simulink model "task3"  (R2023b)
settings: Solver=FixedStepDiscrete  StartTime=0.0  StopTime=10.0  FixedStep=5e-5  RelTol=1e-3
PreLoadFcn:
  | Simulink.defineIntEnumType('windowCommand', {'Off','Speed1','Speed2','Speed3'},[0,1,2,3])
undefined symbols (not defined in the file or in its folder): DiscIntNeverNeededParam, windowCommand
settings Model: Creator=kz1nz0  LastModifiedBy=Zuzia

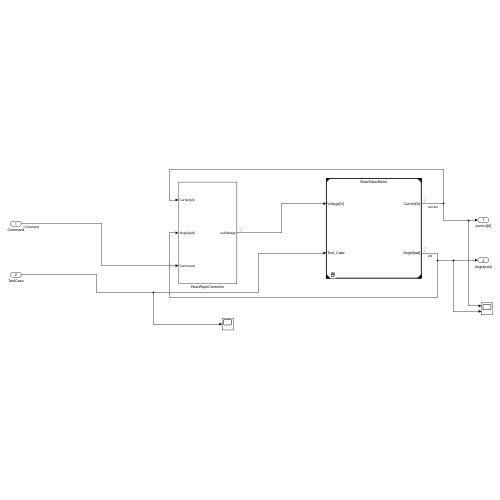
[thumbnail: Simulink's stored preview of the top-level diagram]
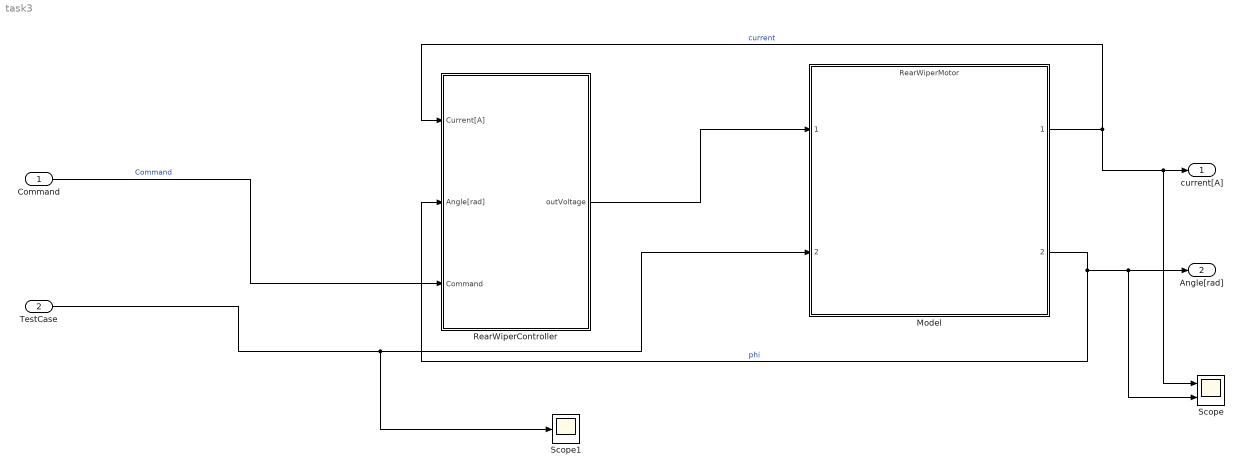
== system task3 ==
  Command : Inport  OutDataTypeStr=Enum: windowCommand
  TestCase : Inport  Port=2  OutDataTypeStr=int8
  Model : ModelReference  ModelNameDialog=RearWiperMotor.slxp  ModelReferenceVersion=19.15  CopyOfModelProtected=on
  RearWiperController : Subsystem
  Scope : Scope  NumInputPorts=2
  Scope1 : Scope
  current[A] : Outport
  Angle[rad] : Outport  Port=2
  wires:
  Command/1 -> RearWiperController/3(Command)  "Command"
  TestCase/1 -> Scope1/1, Model/2
  Model/1 -> Scope/1, current[A]/1, RearWiperController/1(Current[A])  "current"
  Model/2 -> RearWiperController/2(Angle[rad]), Scope/2, Angle[rad]/1  "phi"
  RearWiperController/1(outVoltage) -> Model/1

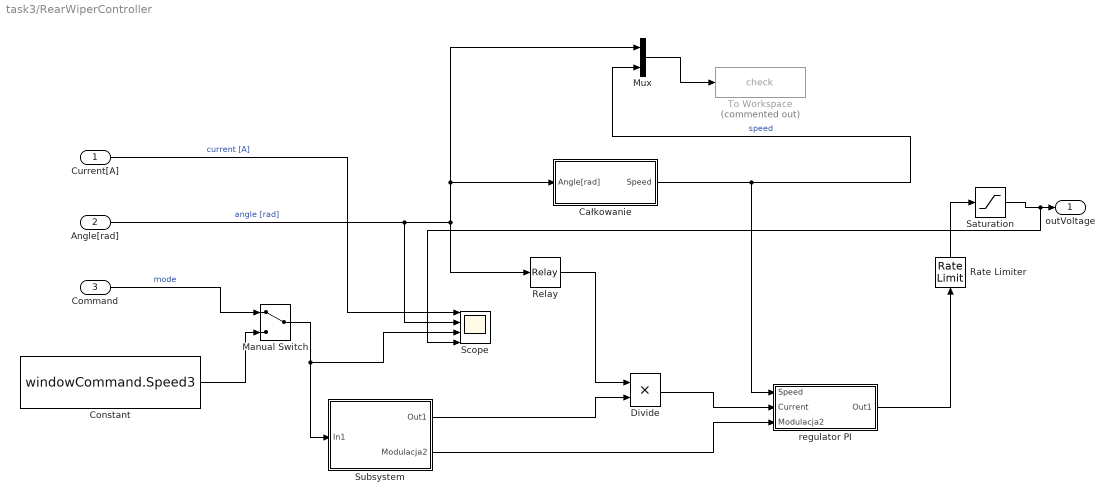
== system task3/RearWiperController ==
  Current[A] : Inport
  Angle[rad] : Inport  Port=2
  Command : Inport  Port=3  OutDataTypeStr=Enum: windowCommand
  Całkowanie : Subsystem
  Constant : Constant  Value=windowCommand.Speed3
  Divide : Product  Inputs=**
  Manual Switch : ManualSwitch
  Mux : Mux  Inputs=2
  Rate Limiter : RateLimiter  RisingSlewLimit=6  FallingSlewLimit=-4  SampleTimeMode=inherited
  Relay : Relay  OnSwitchValue=2.2  OffSwitchValue=0.7  OnOutputValue=-12 * 0.4  OffOutputValue=12 * 0.4
  Saturation : Saturate  UpperLimit=12  LowerLimit=-12
  Scope : Scope  NumInputPorts=4
  Subsystem : Subsystem
  To Workspace : ToWorkspace  Commented=on  VariableName=check  SaveFormat=Timeseries  SampleTime=-1
  regulator PI : Subsystem
  outVoltage : Outport
  wires:
  Angle[rad]/1 -> Scope/2, Całkowanie/1(Angle[rad]), Mux/1, Relay/1  "angle [rad]"
  Current[A]/1 -> Scope/1  "current [A]"
  Saturation/1 -> Scope/4, outVoltage/1
  Command/1 -> Manual Switch/1  "mode"
  Constant/1 -> Manual Switch/2
  Manual Switch/1 -> Scope/3, Subsystem/1(In1)
  Relay/1 -> Divide/1
  Mux/1 -> To Workspace/1
  Całkowanie/1(Speed) -> Mux/2, regulator PI/1(Speed)  "speed"
  Subsystem/1(Out1) -> Divide/2
  Rate Limiter/1 -> Saturation/1
  Divide/1 -> regulator PI/2(Current)
  Subsystem/2(Modulacja2) -> regulator PI/3(Modulacja2)
  regulator PI/1(Out1) -> Rate Limiter/1

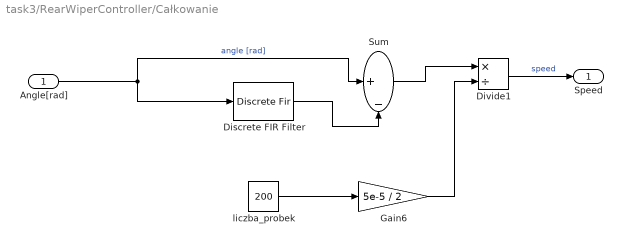
== system task3/RearWiperController/Całkowanie ==
  Angle[rad] : Inport
  Discrete FIR Filter : DiscreteFir  Coefficients=ones(1,200)/200
  Divide1 : Product  Inputs=*/
  Gain6 : Gain  Gain=5e-5 / 2
  Sum : Sum  Inputs=|+-
  liczba_probek : Constant  Value=200
  Speed : Outport
  wires:
  Sum/1 -> Divide1/1
  liczba_probek/1 -> Gain6/1
  Gain6/1 -> Divide1/2
  Angle[rad]/1 -> Sum/1, Discrete FIR Filter/1  "angle [rad]"
  Discrete FIR Filter/1 -> Sum/2
  Divide1/1 -> Speed/1  "speed"

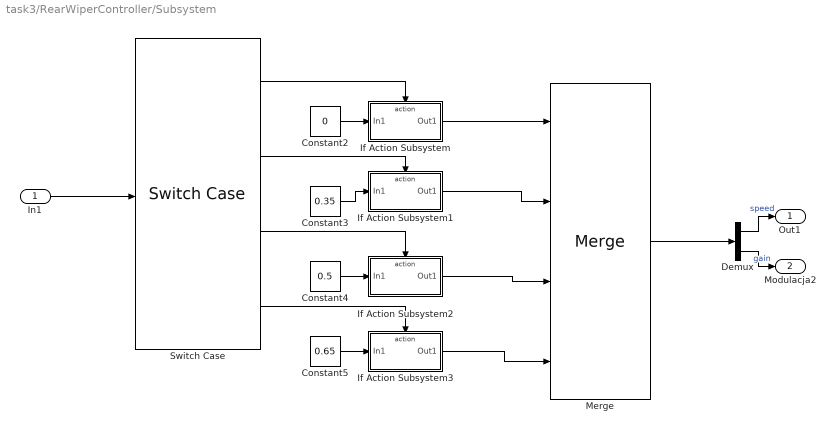
== system task3/RearWiperController/Subsystem ==
  In1 : Inport
  Constant2 : Constant  Value=0
  Constant3 : Constant  Value=0.35
  Constant4 : Constant  Value=0.5
  Constant5 : Constant  Value=0.65
  Demux : Demux  Outputs=2
  If Action Subsystem : Subsystem  TreatAsAtomicUnit=on
  If Action Subsystem1 : Subsystem  TreatAsAtomicUnit=on
  If Action Subsystem2 : Subsystem  TreatAsAtomicUnit=on
  If Action Subsystem3 : Subsystem  TreatAsAtomicUnit=on
  Merge : Merge  Inputs=4
  Switch Case : SwitchCase  CaseConditions={windowCommand.Off,windowCommand.Speed1, windowCommand.Speed2, windowCommand.Speed3}  ShowDefaultCase=off
  Out1 : Outport
  Modulacja2 : Outport  Port=2
  wires:
  In1/1 -> Switch Case/1
  Switch Case/1 -> If Action Subsystem/Action
  Constant2/1 -> If Action Subsystem/1(In1)
  If Action Subsystem/1(Out1) -> Merge/1
  Constant3/1 -> If Action Subsystem1/1(In1)
  If Action Subsystem1/1(Out1) -> Merge/2
  Switch Case/2 -> If Action Subsystem1/Action
  Constant4/1 -> If Action Subsystem2/1(In1)
  If Action Subsystem2/1(Out1) -> Merge/3
  If Action Subsystem3/1(Out1) -> Merge/4
  Constant5/1 -> If Action Subsystem3/1(In1)
  Switch Case/3 -> If Action Subsystem2/Action
  Switch Case/4 -> If Action Subsystem3/Action
  Merge/1 -> Demux/1
  Demux/1 -> Out1/1  "speed"
  Demux/2 -> Modulacja2/1  "gain"

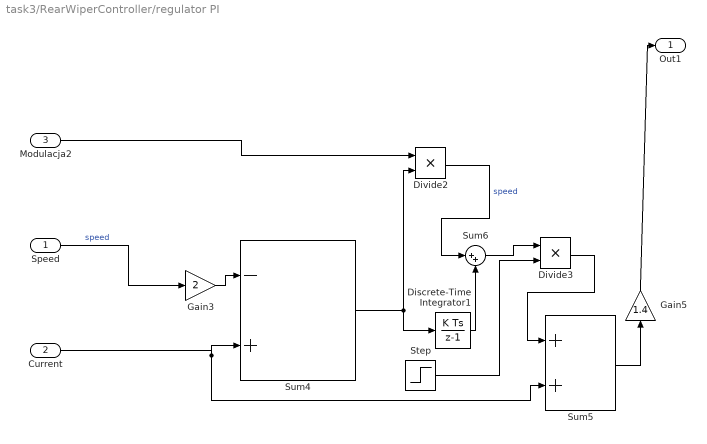
== system task3/RearWiperController/regulator PI ==
  Speed : Inport
  Current : Inport  Port=2
  Modulacja2 : Inport  Port=3
  Discrete-Time Integrator1 : DiscreteIntegrator  gainval=0.02  SampleTime=-1  LimitOutput=on  UpperSaturationLimit=0.1  LowerSaturationLimit=-0.1  ICPrevOutput=DiscIntNeverNeededParam  ICPrevScaledInput=DiscIntNeverNeededParam
  Divide2 : Product  Inputs=**
  Divide3 : Product  Inputs=**
  Gain3 : Gain  Gain=2
  Gain5 : Gain  Gain=1.4
  Step : Step  SampleTime=0
  Sum4 : Sum  Inputs=|-+
  Sum5 : Sum
  Sum6 : Sum  Inputs=|++
  Out1 : Outport
  wires:
  Divide3/1 -> Sum5/1
  Step/1 -> Divide3/2
  Sum6/1 -> Divide3/1
  Speed/1 -> Gain3/1  "speed"
  Gain3/1 -> Sum4/1
  Gain5/1 -> Out1/1
  Modulacja2/1 -> Divide2/1
  Current/1 -> Sum5/2, Sum4/2
  Sum5/1 -> Gain5/1
  Sum4/1 -> Discrete-Time Integrator1/1, Divide2/2
  Divide2/1 -> Sum6/1  "speed"
  Discrete-Time Integrator1/1 -> Sum6/2

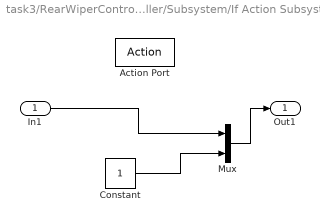
== system task3/RearWiperController/Subsystem/If Action Subsystem ==
  In1 : Inport
  Action Port : ActionPort  ActionPortLabel=case [ Off ]:
  Constant : Constant
  Mux : Mux  Inputs=2
  Out1 : Outport
  wires:
  In1/1 -> Mux/1
  Mux/1 -> Out1/1
  Constant/1 -> Mux/2

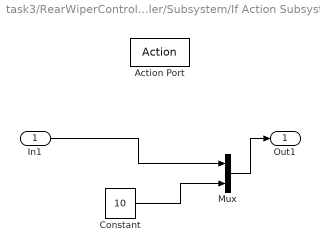
== system task3/RearWiperController/Subsystem/If Action Subsystem1 ==
  In1 : Inport
  Action Port : ActionPort  ActionPortLabel=case [ Speed1 ]:
  Constant : Constant  Value=10
  Mux : Mux  Inputs=2
  Out1 : Outport
  wires:
  In1/1 -> Mux/1
  Constant/1 -> Mux/2
  Mux/1 -> Out1/1

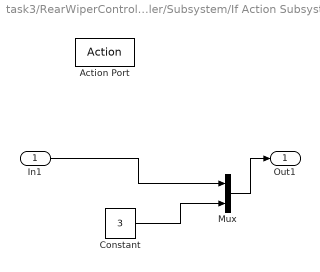
== system task3/RearWiperController/Subsystem/If Action Subsystem2 ==
  In1 : Inport
  Action Port : ActionPort  ActionPortLabel=case [ Speed2 ]:
  Constant : Constant  Value=3
  Mux : Mux  Inputs=2
  Out1 : Outport
  wires:
  In1/1 -> Mux/1
  Constant/1 -> Mux/2
  Mux/1 -> Out1/1

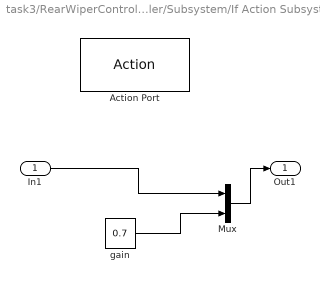
== system task3/RearWiperController/Subsystem/If Action Subsystem3 ==
  In1 : Inport
  Action Port : ActionPort  ActionPortLabel=case [ Speed3 ]:
  Mux : Mux  Inputs=2
  gain : Constant  Value=0.7
  Out1 : Outport
  wires:
  In1/1 -> Mux/1
  gain/1 -> Mux/2
  Mux/1 -> Out1/1
